simulink model "afm_z_simple"  (R2018a)
settings: Solver=VariableStepAuto  StartTime=0.0  StopTime=trun  RelTol=1e-3
undefined symbols (not defined in the file): r
libraries: cstblocks x2
settings Model: Creator=arnold  LastModifiedBy=arnold

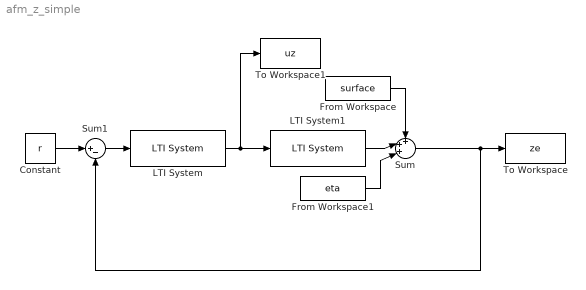
== system afm_z_simple ==
  Constant : Constant  Value=r
  From Workspace : FromWorkspace  VariableName=surface  SampleTime=0
  From Workspace1 : FromWorkspace  VariableName=eta  SampleTime=0
  LTI System : cstblocks/LTI System  sys=Dz  IC=[]
  LTI System1 : cstblocks/LTI System  sys=G1  IC=[]
  Sum : Sum  Inputs=+++|
  Sum1 : Sum  Inputs=|+-
  To Workspace : ToWorkspace  VariableName=ze  SaveFormat=Timeseries  SampleTime=-1
  To Workspace1 : ToWorkspace  VariableName=uz  SaveFormat=Timeseries  SampleTime=-1
  wires:
  From Workspace/1 -> Sum/1
  Sum1/1 -> LTI System/1
  Constant/1 -> Sum1/1
  LTI System/1 -> To Workspace1/1, LTI System1/1
  LTI System1/1 -> Sum/2
  Sum/1 -> To Workspace/1, Sum1/2
  From Workspace1/1 -> Sum/3
